simulink model "Woo_Elizabeth_2_4869"  (R2023b)
settings: Solver=VariableStepAuto  StartTime=0.0  StopTime=0.2  RelTol=1e-6
libraries: spsSeriesRLCBranchLib x5, spsVoltageMeasurementLib x4, spsCurrentMeasurementLib x2, spsDCVoltageSourceLib x1, spsDiodeLib x1, spsGroundLib x1, spsMosfetLib x1, spsPWMGeneratorDCDCLib x1, sps_lib x1
settings Model: Creator=HBeto  LastModifiedBy=rober
settings SolverCC: AlgebraicLoopSolver=TrustRegion
settings DataIOCC: ReturnWorkspaceOutputs=off
settings DebuggingCC: UnconnectedInputMsg=warning  UnconnectedOutputMsg=warning  UnconnectedLineMsg=warning
settings ModelReferenceCC: EnableRefExpFcnMdlSchedulingChecks=on

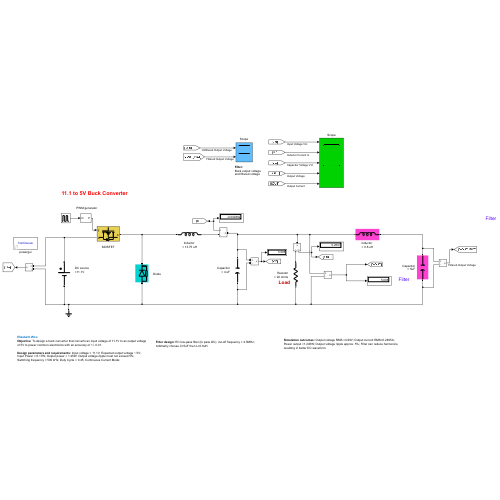
[thumbnail: Simulink's stored preview of the top-level diagram]
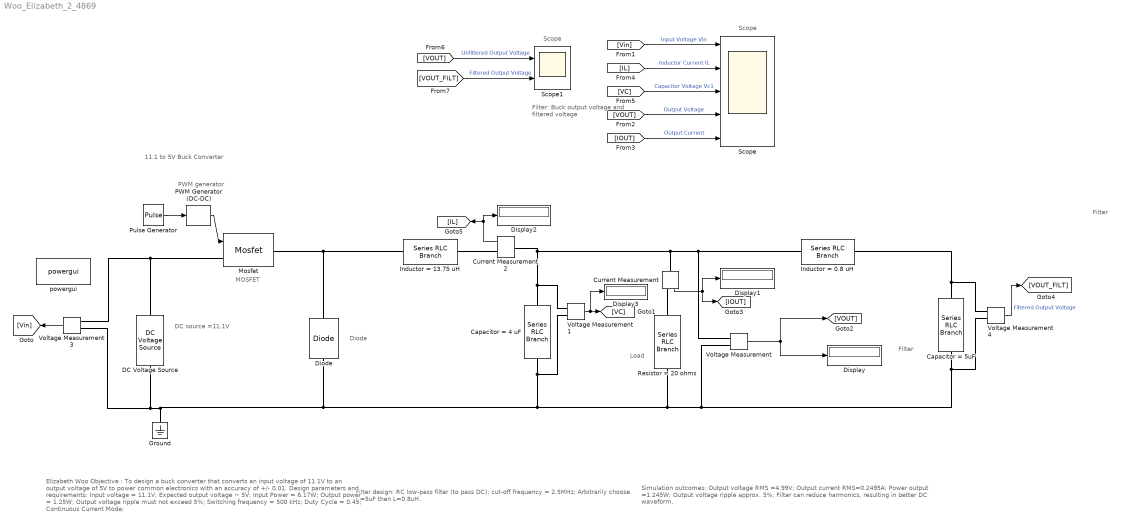
== system Woo_Elizabeth_2_4869 ==
  note: Load
  note: Scope
  note: Simulation outcomes: Output voltage RMS =4.99V; Output current RMS=0.2495A; Power output =1.245W; Output voltage ripple approx. 5%; Filter can reduce harmonics, resulting in better DC waveform.
  note: Filter design: RC low-pass filter (to pass DC); cut-off frequency = 2.5MHz;
      | Arbitrarily choose C=5uF then L=0.8uH.
  note: Filter
  note: DC source
      | =11.1V
  note: Filter:
      | Buck output voltage
      | and filtered voltage
  note: Scope
  note: Elizabeth Woo
      | Objective : To design a buck converter that converts an input voltage of 11.1V to an output voltage of 5V to power common electronics with an accuracy of +/- 0.01.
      |
      | Design parameters and requirements: Input voltage = 11.1V; Expected output voltage ~ 5V; Input Power = 6.17W; Output power = 1.25W; Output voltage ripple must not exceed 5%; Switching frequency = 500 kHz; Duty Cycle = 0.45; Continuous Current Mode;
  note: Diode
  note: MOSFET
  note: PWM generator
  note: 11.1 to 5V Buck Converter
  note: Filter
  Capacitor = 4 uF : spsSeriesRLCBranchLib/Series RLC Branch  LConnTagsString=__new0  RConnTagsString=__new0  BranchType=C  Resistance=0  Inductance=1e-3  SetiL0=off  InitialCurrent=0  Capacitance=3.3e-6  Setx0=off  InitialVoltage=0  Measurements=None
  Capacitor = 5uF : spsSeriesRLCBranchLib/Series RLC Branch  LConnTagsString=__new0  RConnTagsString=__new0  BranchType=C  Resistance=0  Inductance=1e-3  SetiL0=off  InitialCurrent=0  Capacitance=100e-9  Setx0=off  InitialVoltage=0  Measurements=None
  Current Measurement : spsCurrentMeasurementLib/Current Measurement  PhasorSimulation=off  OutputType=Complex  PSBequivalent=0
  Current Measurement2 : spsCurrentMeasurementLib/Current Measurement  PhasorSimulation=off  OutputType=Complex  PSBequivalent=0
  DC Voltage Source : spsDCVoltageSourceLib/DC Voltage Source  Amplitude=11.1  Measurements=None
  Diode : spsDiodeLib/Diode  Ron=0.001  Lon=0  Vf=0  IC=0  UseSnubber=0  Rs=500  Cs=250e-9  Measurements=off
  Display{,1..3} (4 alike) : Display
  Ground : spsGroundLib/Ground  LConnTagsString=a
  Inductor = 0.8 uH : spsSeriesRLCBranchLib/Series RLC Branch  LConnTagsString=__new0  RConnTagsString=__new0  BranchType=L  Resistance=0  Inductance=13.75e-6  SetiL0=off  InitialCurrent=0  Capacitance=0  Setx0=off  InitialVoltage=0  Measurements=None
  Inductor = 13.75 uH : spsSeriesRLCBranchLib/Series RLC Branch  LConnTagsString=__new0  RConnTagsString=__new0  BranchType=L  Resistance=0  Inductance=13.75e-6  SetiL0=off  InitialCurrent=0  Capacitance=0  Setx0=off  InitialVoltage=0  Measurements=None
  Mosfet : spsMosfetLib/Mosfet  Ron=0.1  Lon=0  Rd=0.01  Vfd=0  IC=0  Rs=1e5  Cs=inf  Measurements=off
  PWM Generator (DC-DC) : spsPWMGeneratorDCDCLib/PWM Generator (DC-DC)  Fsw=20000  Ts=0
  Pulse Generator : DiscretePulseGenerator  PulseType=Time based  Period=1/500000  PulseWidth=0.45*100
  Resistor = 20 ohms : spsSeriesRLCBranchLib/Series RLC Branch  LConnTagsString=__new0  RConnTagsString=__new0  BranchType=R  Resistance=20  Inductance=1e-3  SetiL0=off  InitialCurrent=0  Capacitance=1e-6  Setx0=off  InitialVoltage=0  Measurements=None
  Scope : Scope  NumInputPorts=5
  Scope1 : Scope  NumInputPorts=2
  Voltage Measurement{,1,3..4} (4 alike) : spsVoltageMeasurementLib/Voltage Measurement  PhasorSimulation=off  OutputType=Complex  PSBequivalent=0
  powergui : sps_lib/powergui  Priority=1  SimulationMode=Continuous  SampleTime=50e-6  frequency=60  Iterations=50  frequencyindice=0  Pbase=100e6  ErrMax=1e-4  UnitsV=kV  UnitsW=MW  buscounter=0  FunctionMessages=off  echomessages=off  EnableUseOfTLC=off  CurrentSourceSwitches=off  DisableSnubberDevices=off  DisableRonSwitches=off  DisableVfSwitches=off  DisplayEquations=off  AutomaticDiscreteSolvers=off  SolverType=Tustin/Backward Euler (TBE)  Interpol=off  ExternalGateDelay=off  methode=off  Ts=100  x0status=blocks  SPID=on  SwTol=0  HookPort=off  NonlinearTolerance=1e-4  nMaxIteration=100  ContinueOnMaxIteration=off  RestoreLinks=warning  ResistiveCurrentMeasurement=off  Frange=[0:2:500]  Ylog=off  Xlog=on  ShowGrid=off  save=off  variable=ZData  structure=OutputVoltage  ZoomFFT=off  StartTime=0.19  cycles=100  DisplayStyle=1  fundamental=20000  FreqAxis=off  MaxFrequency=100000  frequencyindicesteady=1  RmsSteady=1  display=off
  wires:
  Voltage Measurement/1 -> [VOUT], Display/1
  Current Measurement/1 -> Display1/1, [IOUT]
  [Vin] -> Scope/1  "Input Voltage Vin"
  [IL] -> Scope/2  "Inductor Current IL"
  [VC] -> Scope/3  "Capacitor Voltage Vc1"
  [VOUT] -> Scope/4  "Output Voltage"
  [IOUT] -> Scope/5  "Output Current"
  Current Measurement2/1 -> Display2/1, [IL]
  [VOUT] -> Scope1/1  "Unfiltered Output Voltage"
  PWM Generator (DC-DC)/1 -> Mosfet/1
  [VOUT_FILT] -> Scope1/2  "Filtered Output Voltage"
  Voltage Measurement3/1 -> [Vin]
  Pulse Generator/1 -> PWM Generator (DC-DC)/1
  Voltage Measurement1/1 -> Display3/1, [VC]
  Voltage Measurement4/1 -> [VOUT_FILT]  "Filtered Output Voltage"
  connections:
  Voltage Measurement1/LConn2 -- Capacitor = 4 uF/RConn1 -- Voltage Measurement4/LConn2 -- Capacitor = 5uF/RConn1 -- Voltage Measurement/LConn2 -- Resistor = 20 ohms/RConn1 -- Voltage Measurement3/LConn2 -- DC Voltage Source/LConn1 -- Ground/LConn1 -- Diode/LConn1
  Voltage Measurement/LConn1 -- Inductor = 0.8 uH/LConn1 -- Voltage Measurement1/LConn1 -- Capacitor = 4 uF/LConn1 -- Current Measurement2/LConn1 -- Current Measurement/LConn1
  Resistor = 20 ohms/LConn1 -- Current Measurement/RConn1
  Voltage Measurement3/LConn1 -- Mosfet/LConn1 -- DC Voltage Source/RConn1
  Mosfet/RConn1 -- Inductor = 13.75 uH/LConn1 -- Diode/RConn1
  Current Measurement2/RConn1 -- Inductor = 13.75 uH/RConn1
  Voltage Measurement4/LConn1 -- Inductor = 0.8 uH/RConn1 -- Capacitor = 5uF/LConn1
